simulink model "NEW1"  (Simulink 7.4)
settings: Solver=ode45  StartTime=0.0  StopTime=2.0  RelTol=1e-3
libraries: dspxfrm3 x1, dspsrcs4 x1
settings Model: Creator=jagi20  LastModifiedBy=jagi20

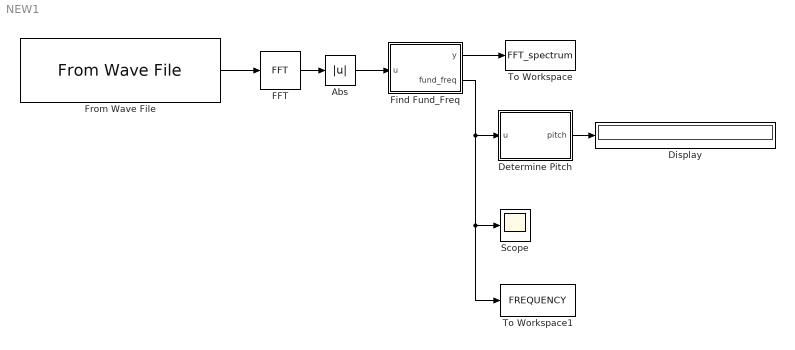
== system NEW1 ==
  Abs : Abs  OutDataType=fixdt(1, 16)  OutScaling=2^0
  Determine Pitch : Stateflow chart
  Display : Display
      settings: Format=long_e
  FFT : dspxfrm3/FFT  DialogController=dspDDGCreate  DialogControllerArgs=DataTag0  CompMethod=Table lookup  TableOpt=NEW  TableOptActive=Speed  BitRevOrder=off  InheritFFTLength=on  FFTLength=64  SkipNorm=off  roundingMode=Floor  overflowMode=off
  Find Fund_Freq : Stateflow chart
  From Wave File : dspsrcs4/From Wave File  FileName=test5_789_8192sample.wav  SamplesPerFrame=8192  MinBufSize=8192  dType=double  bLoop=off  timesToPlay=1  restartMode=immediately after last sample  firstSampleOutput=off  lastSampleOutput=off
  Scope : Scope
  To Workspace : ToWorkspace  VariableName=FFT_spectrum  SampleTime=-1  SaveFormat=Array
  To Workspace1 : ToWorkspace  VariableName=FREQUENCY  SampleTime=-1  SaveFormat=Array
  wires:
  From Wave File/1 -> FFT/1
  FFT/1 -> Abs/1
  Abs/1 -> Find Fund_Freq/1(u)
  Find Fund_Freq/1(y) -> To Workspace/1
  Find Fund_Freq/2(fund_freq) -> Determine Pitch/1(u), Scope/1, To Workspace1/1
  Determine Pitch/1(pitch) -> Display/1

== matlab function Determine Pitch ==
  data: u input double; pitch output double
function pitch = fcn(u)
%#eml

pitch = double(0.0); %initialize pitch value

% AMERICAN STANDARD PITCHES (all in Hz)
% A = 220;
% A1 = 233; % A sharp
% B = 247;
% C = 262; % 'middle C'
% C1 = 277;
% D = 294;
% D1 = 311;
% E = 330;
% F = 349;
% F1 = 370;
% G = 392;
% G1 = 415;

f = round(u); %round to nearest integer

if (f==0) %THIS IS AN ERROR!
    pitch = 9.99999999999999;
elseif (f ~=0)

i=0; %index for iterations of the following loop
while ((f < 212) || (f > 425))
    if f <= 210 %lower octave
        f = 2*f;
        i = i+1;
    elseif (f > 430) 
        f = 0.5*f;
        i = i+1;
    elseif (i > 9999) %prevent inf loop
        break;
    end
end

f = round(f); %make sure it's an integer (again)

if ((212 <= f) && (f <= 226)) 
    pitch = double('A') + .0001*double('0');
elseif ((227 <= f) && (f <= 240)) 
    pitch = double('A') + .0001*double('1');
elseif ((241 <= f) && (f <= 254)) 
    pitch = double('B') + .0001*double('0');
elseif ((255 <= f) && (f <= 269)) 
    pitch = double('C') + .0001*double('0');
elseif ((270 <= f) && (f <= 285)) 
    pitch = double('C') + .0001*double('1');
elseif ((286 <= f) && (f <= 302)) 
    pitch = double('D') + .0001*double('0');
elseif ((303 <= f) && (f <= 320)) 
    pitch = double('D') + .0001*double('1');
elseif ((321 <= f) && (f <= 339)) 
    pitch = double('E') + .0001*double('0');
elseif ((340 <= f) && (f <= 359))
    pitch = double('F') + .0001*double('0');
elseif ((360 <= f) && (f <= 381))
    pitch = double('F') + .0001*double('1');
elseif ((382 <= f) && (f <= 403)) 
    pitch = double('G') + .0001*double('0');
elseif ((404 <= f) && (f <= 425))
    pitch = double('G') + .0001*double('1');
end

end

== matlab function Find Fund_Freq ==
  data: u input double; y output double; fund_freq output double
function [y,fund_freq] = fcn(u)
%#eml

y = u;

value = max(u);
a = find(u==value,1) -1;
fund_freq = a(1,1); %a scalar
